simulink model "SortierAlgorithmusVirtuelleTestumgebung"  (R2018b)
settings: Solver=FixedStepDiscrete  StartTime=0.0  StopTime=100  RelTol=1e-3  EnableMultiTasking=on
undefined symbols (not defined in the file): sigbuilder_block
libraries: commrandsrc3 x1
settings Model: ExtModeTrigDuration=8  Creator=Nici  LastModifiedBy=User
settings SolverCC: AutoInsertRateTranBlk=on
settings OptimizationCC: DefaultUnderspecifiedDataType=single  EnhancedBackFolding=on  PassReuseOutputArgsAs=Individual arguments  MaxStackSize=512  OptimizeBlockOrder=speed  DifferentSizesBufferReuse=on  OptimizationCustomize=off
settings DebuggingCC: ParameterTunabilityLossMsg=error  UnderSpecifiedDataTypeMsg=warning
settings HardwareCC: ProdBitPerChar=16  ProdBitPerInt=16  ProdBitPerPointer=32  ProdBitPerSizeT=32  ProdBitPerPtrDiffT=32  ProdLargestAtomicInteger=Integer  ProdLargestAtomicFloat=None  ProdWordSize=16  ProdLongLongMode=on  ProdHWDeviceType=Texas Instruments->C2000
settings SFSimCC: MATLABDynamicMemAlloc=off
settings RTWCC: SystemTargetFile=ert.tlc  HardwareBoard=TI Delfino F2833x  TemplateMakefile=ert_default_tmf  GenerateReport=on  Toolchain=Texas Instruments Code Composer Studio (C2000)  IncludeHyperlinkInReport=on  LaunchReport=on  GenerateTraceInfo=on  GenerateTraceReport=on  GenerateTraceReportSl=on  GenerateTraceReportSf=on  GenerateTraceReportEml=on
settings CodeAppCC: ForceParamTrailComments=on  IgnoreCustomStorageClasses=off  OperatorAnnotations=on  SimulinkDataObjDesc=on  SFDataObjDesc=on  InsertBlockDesc=on
settings ERTTargetCC: CodeReplacementLibrary=TI C28x  SupportContinuousTime=on

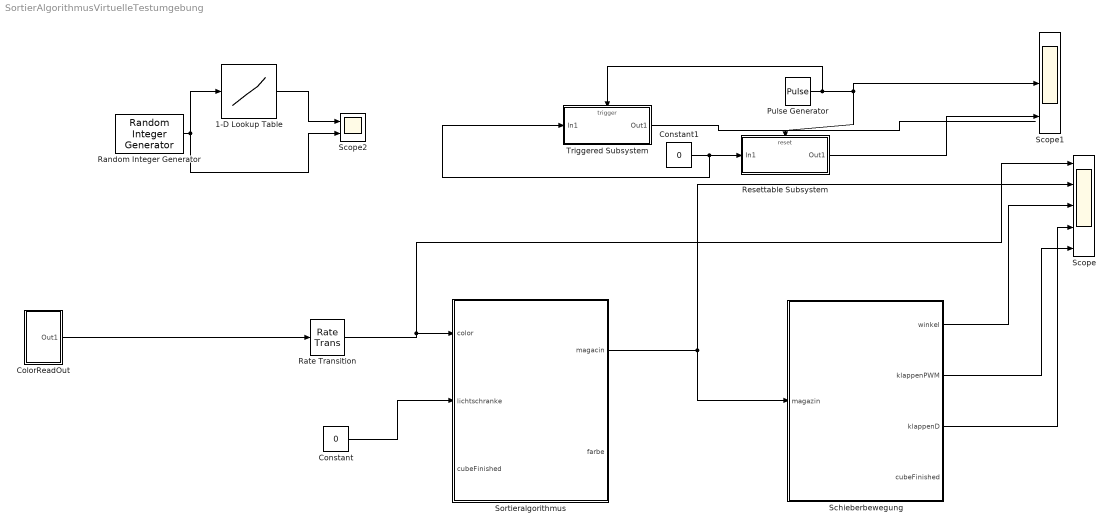
== system SortierAlgorithmusVirtuelleTestumgebung ==
  1-D Lookup Table : Lookup_n-D  NumberOfTableDimensions=1  BreakpointsForDimension1=[0,1,2,3,4,5,6]  Table=[-440,-295,-170,-40,85,220,430]  InternalRulePriority=Speed  RndMeth=Simplest  InputSameDT=on
  ColorReadOut : Subsystem
  Constant : Constant  Value=0
  Constant1 : Constant  Value=0
  Pulse Generator : DiscretePulseGenerator  PulseType=Time based  Period=10  PulseWidth=5
  Random Integer Generator : commrandsrc3/Random Integer Generator  SetSize=7  SeedSource=Auto  Seed=0  SampleTime=1  SamplesPerFrame=1  OutputDataType=double  SimulateUsing=Interpreted execution
  Rate Transition : RateTransition  InitialCondition=1  OutPortSampleTime=0.01
  Resettable Subsystem : Subsystem  TreatAsAtomicUnit=on
  Schieberbewegung : Stateflow chart  TreatAsAtomicUnit=on
  Scope : Scope  NumInputPorts=5
  Scope1 : Scope  NumInputPorts=3
  Scope2 : Scope  NumInputPorts=2
  Sortieralgorithmus : Stateflow chart  TreatAsAtomicUnit=on
  Triggered Subsystem : Subsystem  TreatAsAtomicUnit=on
  wires:
  Constant/1 -> Sortieralgorithmus/2(lichtschranke)
  ColorReadOut/1(Out1) -> Rate Transition/1
  Rate Transition/1 -> Scope/1, Sortieralgorithmus/1(color)
  Sortieralgorithmus/1(magacin) -> Schieberbewegung/1(magazin), Scope/2
  Schieberbewegung/1(winkel) -> Scope/3
  Schieberbewegung/3(klappenD) -> Scope/4
  Schieberbewegung/2(klappenPWM) -> Scope/5
  Pulse Generator/1 -> Resettable Subsystem/Reset, Scope1/2, Triggered Subsystem/Trigger
  Resettable Subsystem/1(Out1) -> Scope1/3
  Constant1/1 -> Triggered Subsystem/1(In1), Resettable Subsystem/1(In1)
  Triggered Subsystem/1(Out1) -> ?
  Random Integer Generator/1 -> Scope2/2, 1-D Lookup Table/1
  1-D Lookup Table/1 -> Scope2/1

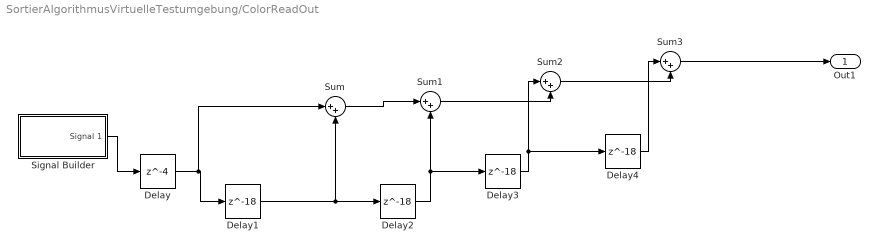
== system SortierAlgorithmusVirtuelleTestumgebung/ColorReadOut ==
  Delay : Delay  DelayLength=4  SampleTime=1
  Delay{1..4} (4 alike) : Delay  DelayLength=18  SampleTime=1
  Signal Builder : Subsystem  Tag=STV Subsys  LoadFcn=sigbuilder_block('load');  StartFcn=sigbuilder_block('start');  StopFcn=sigbuilder_block('stop');  ClipboardFcn=sigbuilder_block('clipboard');  mask(Sigbuilder block){tuvar=[0:10]}
      mask help: Simulink:masks:SigbuilderBlock_MD
      mask init:
      | if ~strcmp(get_param(bdroot(gcbh),'SimulationStatus'),'stopped') tuvar = sigbuilder_block('maskInit'); end
      settings: CopyFcn=sigbuilder_block('copy');  DeleteFcn=sigbuilder_block('delete');  ModelCloseFcn=sigbuilder_block('modelClose');  PreSaveFcn=sigbuilder_block('preSave');  PauseFcn=sigbuilder_block('pause');  ContinueFcn=sigbuilder_block('continue');  NameChangeFcn=sigbuilder_block('namechange');  OpenFcn=sigbuilder_block('open',[404.625 178.125 550.5 364.5 ]);  CloseFcn=sigbuilder_block('close');
      mask Display: plot(0, 0, 100, 100,[2, 2, 32, 32, 2], [68, 8, 8, 68, 68],[32, 2], [38, 38], [32, 19, 2],[53, 60, 44], [32, 17, 17, 2],[16, 16, 31, 31]);txt = getActiveGroup(gcbh);text(2, 100, txt,'verticalAlignment', 'top');
  Sum{,1..3} (4 alike) : Sum  Inputs=|++
  Out1 : Outport
  wires:
  Delay3/1 -> Delay4/1, Sum2/1
  Sum/1 -> Sum1/1
  Signal Builder/1(Signal 1) -> Delay/1
  Sum1/1 -> Sum2/2
  Delay2/1 -> Delay3/1, Sum1/2
  Delay1/1 -> Delay2/1, Sum/2
  Delay/1 -> Sum/1, Delay1/1
  Sum3/1 -> Out1/1
  Sum2/1 -> Sum3/2
  Delay4/1 -> Sum3/1

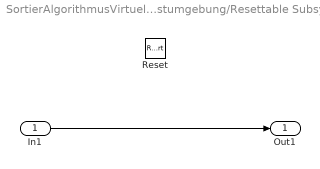
== system SortierAlgorithmusVirtuelleTestumgebung/Resettable Subsystem ==
  In1 : Inport
  Reset : ResetPort  DisableCoverage=on
  Out1 : Outport
  wires:
  In1/1 -> Out1/1

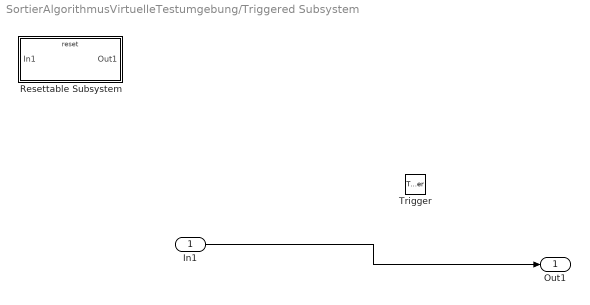
== system SortierAlgorithmusVirtuelleTestumgebung/Triggered Subsystem ==
  In1 : Inport
  Trigger : TriggerPort  VariantControl=Variant  StatesWhenEnabling=reset  OutputDataType=double
  Resettable Subsystem : Subsystem  TreatAsAtomicUnit=on
  Out1 : Outport
  wires:
  In1/1 -> Out1/1

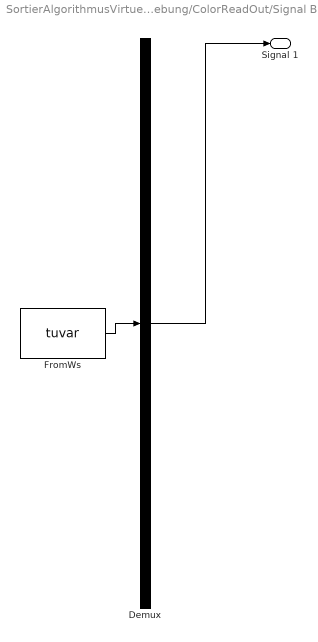
== system SortierAlgorithmusVirtuelleTestumgebung/ColorReadOut/Signal Builder ==
  Demux : Demux  Tag=STV Demux  Outputs=1
  FromWs : FromWorkspace  Tag=STV FromWs  VariableName=tuvar  SampleTime=0
      SigBuilderData=|
      | common.afterFinalStr = 'Extrapolate'
      | common.sampleTime = 0
      | dataSet.timeRange = [0 30]
      | dataSet.name = 'Group 1'
      | sbobj.Groups.Name = 'Group 1'
      | sbobj.Groups.Signals.Name = 'Signal 1'
      | sbobj.Groups.Signals.XData = [0 1 1 3 3 4 4 6 6 7 7 9 9 10 10 12 12 13 13 15 15 16 16 21.5 21.5 23.3 24.55 25.55 26.7 28.05 30]
      | sbobj.Groups.Signals.YData = [1800 1800 0 0 1800 1800 0 0 200 200 0 0 200 200 0 0 1800 1800 0 0 1800 1800 0 0 0 0 0 0 0 0 0]
      | sbobj.Groups.TimeRange = [0 30]
  Signal 1 : Outport  Tag=STV Outport
  wires:
  Demux/1 -> Signal 1/1
  FromWs/1 -> Demux/1

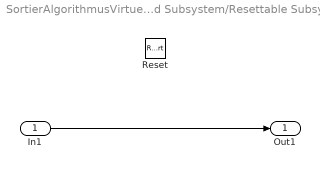
== system SortierAlgorithmusVirtuelleTestumgebung/Triggered Subsystem/Resettable Subsystem ==
  In1 : Inport
  Reset : ResetPort  DisableCoverage=on
  Out1 : Outport
  wires:
  In1/1 -> Out1/1

== stateflow chart SortierAlgorithmusVirtuelleTestumgebung/Schieberbewegung ==
  state firstEntry
    entry: winkel = 300;
  note: StartWinkel, da SChieber nicht in Mitte stehen darf am Anfang. 5 Sekunden Zeit um das Bord einzuschalten
  state waitForCube
    cubeFinished = 1;
  state closeKlappe
    klappenD = 0;
  note: Schwarzer Stein
  state goToZero7
    winkel = 0;
    cubeFinished = 0;
  state goToZero1
    winkel = 0;
    cubeFinished = 0;
  state goToZero2
    winkel = 0;
    cubeFinished = 0;
  state goToZero3
    winkel = 0;
    cubeFinished = 0;
  state goToZero4
    winkel = 0;
    cubeFinished = 0;
  state goToZero5
    winkel = 0;
    cubeFinished = 0;
  state goToZero6
    winkel = 0;
    cubeFinished = 0;
  state wait6
    klappenPWM = 0;
  state wait2
    klappenPWM = 0;
  state wait
    klappenPWM = 0;
  state wait1
    klappenPWM = 0;
  state wait3
    klappenPWM = 0;
  state wait4
    klappenPWM = 0;
  state wait5
    klappenPWM = 0;
  state Linksdrehen5
    entry: winkel = 430;
  state Linksdrehen
    entry: winkel = -295;
  state Linksdrehen1
    entry: winkel = -170;
  state Linksdrehen2
    entry: winkel = -40;
  state Linksdrehen3
    entry: winkel = 85;
  state Linksdrehen4
    entry: winkel = 220;
  state Rechtsdrehen
    entry: winkel = -440;
  state openKlappe
    klappenPWM = 50;
    klappenD = 1;
  (default) -> firstEntry
  firstEntry -> waitForCube : [after(3,sec)]
  closeKlappe -> waitForCube
  waitForCube -> waitForCube [order 8] : [after(0.5,sec)]{klappenPWM = 0;}
  waitForCube -> goToZero1 [order 1] : [magazin == 0]
  waitForCube -> goToZero2 [order 2] : [magazin == 1]
  waitForCube -> goToZero3 [order 7] : [magazin == 2]
  waitForCube -> goToZero4 [order 6] : [magazin == 3]
  waitForCube -> goToZero5 [order 5] : [magazin == 4]
  waitForCube -> goToZero6 [order 4] : [magazin == 5]
  waitForCube -> goToZero7 [order 3] : [magazin == 6]
  openKlappe -> closeKlappe : [after(0.7, sec)]
  goToZero7 -> wait6 : [after(1,sec)]
  goToZero1 -> wait2 : [after(1,sec)]
  goToZero2 -> wait : [after(1,sec)]
  goToZero3 -> wait1 : [after(1,sec)]
  goToZero4 -> wait3 : [after(1,sec)]
  goToZero5 -> wait4 : [after(1,sec)]
  goToZero6 -> wait5 : [after(1,sec)]
  wait6 -> Linksdrehen5 : [after(0.1, sec)]
  wait1 -> Linksdrehen1 : [after(0.1, sec)]
  wait3 -> Linksdrehen2 : [after(0.1, sec)]
  wait4 -> Linksdrehen3 : [after(0.1, sec)]
  wait5 -> Linksdrehen4 : [after(0.1, sec)]
  wait2 -> Rechtsdrehen : [after(0.1, sec)]
  wait -> Linksdrehen : [after(0.1,sec)]
  Linksdrehen5 -> openKlappe : [after(1,sec)]
  Rechtsdrehen -> openKlappe : [after(1,sec)]
  Linksdrehen4 -> openKlappe : [after(1,sec)]
  Linksdrehen3 -> openKlappe : [after(1,sec)]
  Linksdrehen2 -> openKlappe : [after(1,sec)]
  Linksdrehen1 -> openKlappe : [after(1,sec)]
  Linksdrehen -> openKlappe : [after(1,sec)]
  data: magazin input; winkel output; klappenPWM output; klappenD output; cubeFinished output

== stateflow chart SortierAlgorithmusVirtuelleTestumgebung/Sortieralgorithmus ==
  state setupVariable
    m0 = 0;
    m1 = 0;
    m2 = 0;
    m3 = 0;
    m4 = 0;
    m5 = 0;
    m6 = 0;
    m0_LC = 0;
    m1_LC = 0;
    m2_LC = 0;
    m3_LC = 0;
    m4_LC = 0;
    m5_LC = 0;
    m6_LC = 0;
    magacin = -1;
  note: Motor fahre Position Mitte an
  note: 1 ist Code for Blue, 2 is Code for Red, 3 is Code for Black, 0 is empty
  state cubeLoaded
    magacin = -1;
    farbe = -1;
  state SchrankeAktiviert
  state BlueCube
    entry: magacin = findPlaceForBlue();
    farbe = 1;
  state Black
    magacin = 6;
    farbe = 2;
  state RedCube
    entry: magacin = findPlaceForRed();
    farbe = 0;
  state DetectedCube
    magacin = -1;
  setupVariable -> cubeLoaded
  (default) -> setupVariable
  DetectedCube -> cubeLoaded
  cubeLoaded -> SchrankeAktiviert : [lichtschranke < 400]
  SchrankeAktiviert -> BlueCube [order 3] : [((color >= 1000) && (color <= 2050)) ]
  SchrankeAktiviert -> RedCube [order 2] : [(color > 0) && (color < 1000)]
  SchrankeAktiviert -> Black [order 1] : [(color > 2050)]
  BlueCube -> DetectedCube : [after(1.5,sec)]
  Black -> DetectedCube : [after(1.5,sec)]
  RedCube -> DetectedCube : [after(1.5,sec)]
  data: magacinOut function_output; magacinOut function_output; color input; m6 local; m0_LC local; m3_LC local; m2_LC local; m5_LC local; m1_LC local; m6_LC local; m4_LC local; magacin output; farbe output; lichtschranke input; m0 local; m1 local int32; m2 local int32; m3 local; m4 local; m5 local; cubeFinished input
  function magacinOut  = findPlaceForRed:
    | function magacinOut  = findPlaceForRed
    | 
    | %1 ist Code for Blue, 2 is Code for Red, 3 is Code for Black, 0 is empty
    | if((m1 == 0) || ((m1_LC == 1)&& (m1 < 5)))
    |             magacinOut = 1;
    |             m1 = m1 + 1;
    |             m1_LC = 2;
    | elseif (((m2_LC == 1) && (m2 < 5)))
    |             magacinOut = 2;
    |             m2 = m2 + 1; 
    |             m2_LC = 2;
    | elseif ((m0 < 5) && (m0 > 0))
    |             magacinOut = 0;
    |             m0 = m0 + 1;
    |             m0_LC = 2;
    | else 
    |             magacinOut = 3;
    |             m3 = m3 + 1;
    |             m3_LC = 2;
    | end
  function magacinOut  = findPlaceForBlue:
    | function magacinOut  = findPlaceForBlue
    | 
    | %1 ist Code for Blue, 2 is Code for Red, 3 is Code for Black, 0 is empty
    | magacinOut = 5;
    | if(m0 == 0)  
    |             magacinOut = 0;
    |             m0 = (m0 + 1);
    |             m0_LC = 1;
    | elseif ((m2 == 0) || (m2_LC == 2 && m2 < 5))
    |             magacinOut = 2;
    |             m2 = m2 + 1; 
    |             m2_LC = 1;
    | elseif ((m1_LC == 2) && (m1 < 5))
    |             magacinOut = 1;
    |             m1 = m1 + 1;
    |             m1_LC = 1;
    | elseif (m3 < 5)
    |             magacinOut = 3;
    |             m3 = (m3 + 1);
    | elseif (m4 < 5)
    |             magacinOut = 4;
    |             m4 = (m4 + 1);
    | %else
    |  %           magacinOut = 5;
    |   %          m5 = m5 + 1;
    | end
